simulink model "FCW_ROS_V1"  (R2022a)
settings: Solver=ode1  StartTime=0.0  StopTime=50  FixedStep=1  RelTol=1e-3
undefined symbols (not defined in the file): ACC, sigbuilder_block, speedController
libraries: slpidlib x5, simulink x2, robotlib x2
settings Model: NumberOfSteps=10  Creator=Kunj Patel  LastModifiedBy=dorleco
settings SolverCC: AlgebraicLoopSolver=TrustRegion
settings DebuggingCC: UnconnectedInputMsg=warning  UnconnectedOutputMsg=warning  UnconnectedLineMsg=warning  SFMachineParentedDataDiag=warning
settings SFSimCC: SimParseCustomCode=off
settings RTWCC: DLArmComputeVersion=19.05

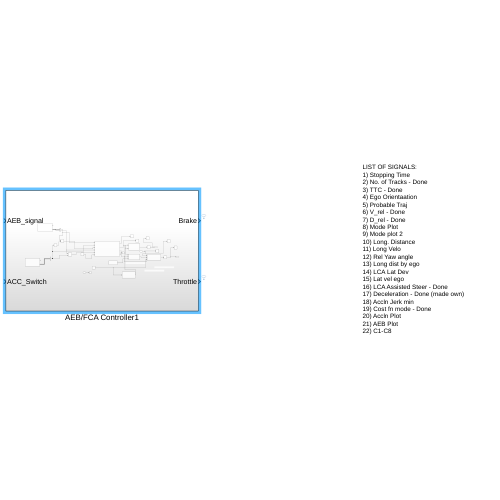
[thumbnail: Simulink's stored preview of the top-level diagram]
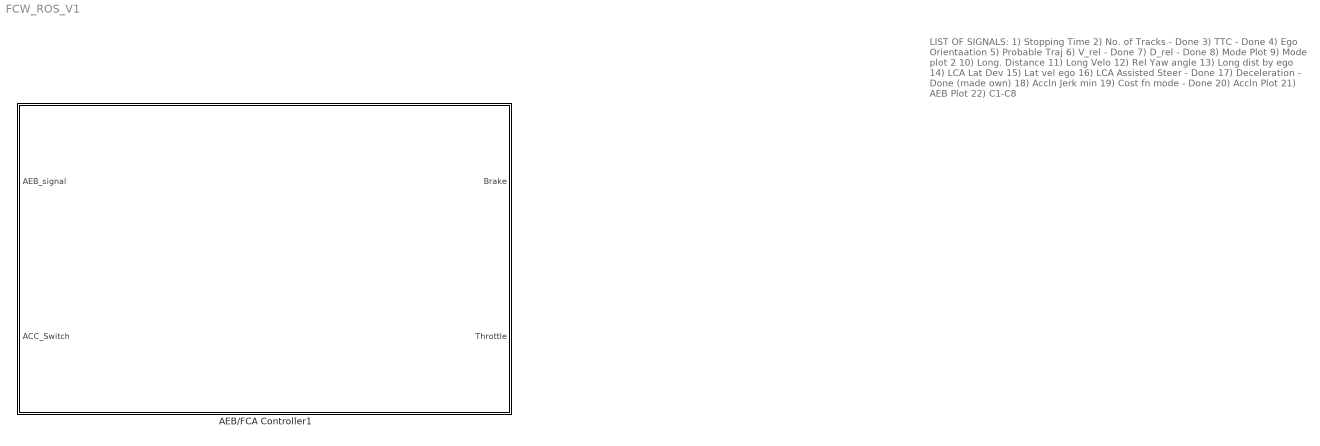
== system FCW_ROS_V1 ==
  note: LIST OF SIGNALS:
      | 1) Stopping Time
      | 2) No. of Tracks - Done
      | 3) TTC - Done
      | 4) Ego Orientaation
      | 5) Probable Traj
      | 6) V_rel - Done
      | 7) D_rel - Done
      | 8) Mode Plot
      | 9) Mode plot 2
      | 10) Long. Distance
      | 11) Long Velo
      | 12) Rel Yaw angle
      | 13) Long dist by ego
      | 14) LCA Lat Dev
      | 15) Lat vel ego
      | 16) LCA Assisted Steer - Done
      | 17) Deceleration - Done (made own)
      | 18) Accln Jerk min
      | 19) Cost fn mode - Done
      | 20) Accln Plot
      | 21) AEB Plot
      | 22) C1-C8
  AEB/FCA Controller1 : Subsystem

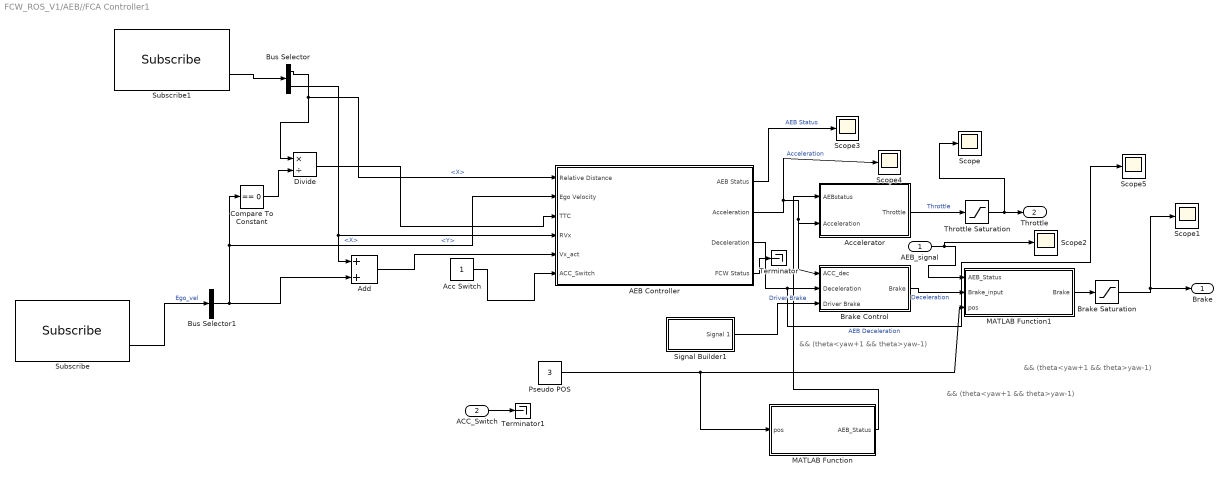
== system FCW_ROS_V1/AEB//FCA Controller1 ==
  note: && (theta<yaw+1 && theta>yaw-1)
  note: && (theta<yaw+1 && theta>yaw-1)
  note: && (theta<yaw+1 && theta>yaw-1)
  AEB_signal : Inport
  ACC_Switch : Inport  Port=2
  AEB Controller : Subsystem
  Acc Switch : Constant
  Accelerator : Subsystem
  Add : Sum
  Brake Control : Subsystem
  Brake Saturation : Saturate  UpperLimit=8  LowerLimit=0
  Bus Selector : BusSelector  OutputSignals=X,Y
  Bus Selector1 : BusSelector  OutputSignals=Twist.Twist.Linear.X
  Compare To Constant : simulink/Logic and Bit Operations/Compare To Constant  relop===  const=0  OutDataTypeStr=boolean
  Divide : Product  Inputs=*/
  MATLAB Function : MATLAB Function  TreatAsAtomicUnit=on
  MATLAB Function1 : MATLAB Function  TreatAsAtomicUnit=on
  Pseudo POS : Constant  Value=3
  Scope{,1..5} (6 alike) : Scope
  Signal Builder1 : Subsystem  Tag=STV Subsys  LoadFcn=sigbuilder_block('load');  StartFcn=sigbuilder_block('start');  StopFcn=sigbuilder_block('stop');  ClipboardFcn=sigbuilder_block('clipboard');  mask(Sigbuilder block){tuvar=[0:10]}
      mask help: Simulink:masks:SigbuilderBlock_MD
      mask init:
      | if ~strcmp(get_param(bdroot(gcbh),'SimulationStatus'),'stopped') tuvar = sigbuilder_block('maskInit'); end
      settings: CopyFcn=sigbuilder_block('copy');  DeleteFcn=sigbuilder_block('delete');  ModelCloseFcn=sigbuilder_block('modelClose');  PreSaveFcn=sigbuilder_block('preSave');  PauseFcn=sigbuilder_block('pause');  ContinueFcn=sigbuilder_block('continue');  NameChangeFcn=sigbuilder_block('namechange');  OpenFcn=sigbuilder_block('open',[302 88 550.5 362.5 ]);  CloseFcn=sigbuilder_block('close');
      mask Display: plot(0, 0, 100, 100,[2, 2, 32, 32, 2], [68, 8, 8, 68, 68],[32, 2], [38, 38], [32, 19, 2],[53, 60, 44], [32, 17, 17, 2],[16, 16, 31, 31]);txt = getActiveGroup(gcbh);text(2, 100, txt,'verticalAlignment', 'top');
  Subscribe : robotlib/Subscribe  topicSource=Select from ROS network  topic=/carla/ego_vehicle/odometry  messageType=nav_msgs/Odometry  SampleTime=1  legacyBusStruct=off  messageQueueLength=1
  Subscribe1 : robotlib/Subscribe  topicSource=Select from ROS network  topic=/perception/FCW  messageType=geometry_msgs/Point  SampleTime=1  legacyBusStruct=off  messageQueueLength=1
  Terminator : Terminator
  Terminator1 : Terminator
  Throttle Saturation : Saturate  UpperLimit=1.3  LowerLimit=0
  Brake : Outport
  Throttle : Outport  Port=2
  wires:
  Signal Builder1/1(Signal 1) -> Brake Control/3(Driver Brake)  "Driver Brake"
  AEB Controller/3(Deceleration) -> Scope5/1, Brake Control/2(Deceleration)  "AEB Deceleration"
  Accelerator/1(Throttle) -> Throttle Saturation/1  "Throttle"
  Throttle Saturation/1 -> Scope/1, Throttle/1
  Brake Saturation/1 -> Scope1/1, Brake/1
  AEB Controller/2(Acceleration) -> Scope4/1, Brake Control/1(ACC_dec), Accelerator/2(Acceleration)  "Acceleration"
  Divide/1 -> AEB Controller/3(TTC)
  AEB Controller/4(FCW Status) -> Terminator/1
  MATLAB Function1/1(Brake) -> Brake Saturation/1
  Brake Control/1(Brake) -> MATLAB Function1/2(Brake_input)  "Deceleration"
  AEB_signal/1 -> MATLAB Function1/1(AEB_Status), Scope2/1
  AEB Controller/1(AEB Status) -> Scope3/1  "AEB Status"
  MATLAB Function/1(AEB_Status) -> Accelerator/1(AEBstatus)
  ACC_Switch/1 -> Terminator1/1
  Acc Switch/1 -> AEB Controller/6(ACC_Switch)
  Pseudo POS/1 -> MATLAB Function1/3(pos), MATLAB Function/1(pos)
  Subscribe1/2 -> Bus Selector/1
  Subscribe/2 -> Bus Selector1/1  "Ego_vel"
  Bus Selector/1 -> AEB Controller/1(Relative Distance), Divide/1  "<X>"
  Bus Selector1/1 -> AEB Controller/2(Ego Velocity), Compare To Constant/1, Add/2  "<X>"
  Bus Selector/2 -> Add/1, AEB Controller/4(RVx)  "<Y>"
  Add/1 -> AEB Controller/5(Vx_act)
  Compare To Constant/1 -> Divide/2

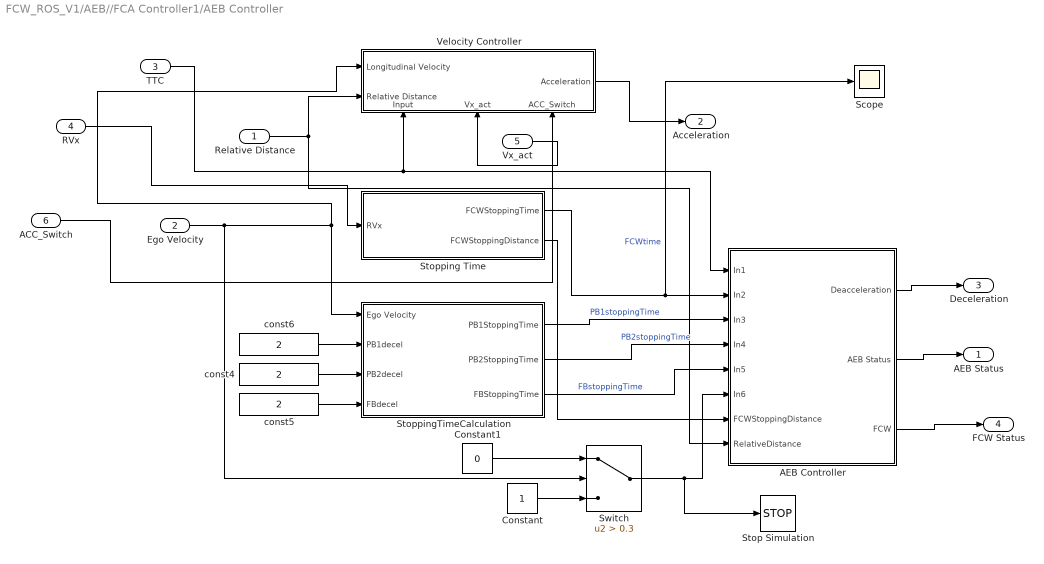
== system FCW_ROS_V1/AEB//FCA Controller1/AEB Controller ==
  Relative Distance : Inport
  Ego Velocity : Inport  Port=2
  TTC : Inport  Port=3
  RVx : Inport  Port=4
  Vx_act : Inport  Port=5
  ACC_Switch : Inport  Port=6
  AEB Controller : Subsystem
  Constant : Constant
  Constant1 : Constant  Value=0
  Scope : Scope
  Stop Simulation : Stop
  Stopping Time : Subsystem
  StoppingTimeCalculation : Subsystem
  Switch : Switch  Criteria=u2 > Threshold  Threshold=0.3  SaturateOnIntegerOverflow=off  InputSameDT=off
  Velocity Controller : Subsystem
      settings: PortSchema="{\"entries\":[{\"content\":{\"sides\":[{\"content\":{\"connectorIds\":[\"In1\",\"In2\"]},\"type\":\"ConnectorPlacement.EquallySpacedRectSide\",\"uuid\":\"796c06ee-5e3e-4c70-89bb-3872b2b2fec3\"},{\"content\":{\"connectorIds\":[\"Out1\"],\"side\":\"RIGHT\"},\"type\":\"ConnectorPlacement.EquallySpacedRectSide\",\"uuid\":\"23e41fbd-8b20-4aaf-a094-11b66cab9187\"},{\"content\":{\"connectorIds\":[],\"side\":\"TOP\"},\"type\":\"ConnectorPlacement.EquallySpacedRectSide\",\"uuid\":\"26342e9d-9e9e-43cc-a4c5-bfbf2895aede\"},{\"content\":{\"connectorIds\":[\"In3\",\"In4\",\"In5\"],\"side\":\"BOTTOM\"},\"type\":\"ConnectorPlacement.EquallySpacedRectSide\",\"uuid\":\"03d34232-b2fb-4d0e-a887-0a4704da0eeb\"}]},\"type\":\"ConnectorPlacement.EquallySpacedConnector\",\"uuid\":\"68d7bb64-97bc-4384-b049-e1fd777b4ed3\"}],\"packageUris\":[\"http://schema.mathworks.com/mf0/Connector/R2020b\"],\"version\":\"1.0\"}"
  const4 : Constant  Value=2  SampleTime=-1
  const5 : Constant  Value=2  SampleTime=-1
  const6 : Constant  Value=2  SampleTime=-1
  AEB Status : Outport  VectorParamsAs1DForOutWhenUnconnected=off
  Acceleration : Outport  Port=2  VectorParamsAs1DForOutWhenUnconnected=off
  Deceleration : Outport  Port=3  VectorParamsAs1DForOutWhenUnconnected=off
  FCW Status : Outport  Port=4  VectorParamsAs1DForOutWhenUnconnected=off
  wires:
  Relative Distance/1 -> AEB Controller/8(RelativeDistance), Velocity Controller/2(Relative Distance)
  const5/1 -> StoppingTimeCalculation/4(FBdecel)
  Stopping Time/1(FCWStoppingTime) -> Scope/1, AEB Controller/2(In2)  "FCWtime"
  const4/1 -> StoppingTimeCalculation/3(PB2decel)
  const6/1 -> StoppingTimeCalculation/2(PB1decel)
  Velocity Controller/1(Acceleration) -> Acceleration/1
  AEB Controller/2(AEB Status) -> AEB Status/1
  AEB Controller/1(Deacceleration) -> Deceleration/1
  AEB Controller/3(FCW) -> FCW Status/1
  StoppingTimeCalculation/3(FBStoppingTime) -> AEB Controller/5(In5)  "FBstoppingTime"
  StoppingTimeCalculation/2(PB2StoppingTime) -> AEB Controller/4(In4)  "PB2stoppingTime"
  StoppingTimeCalculation/1(PB1StoppingTime) -> AEB Controller/3(In3)  "PB1stoppingTime"
  TTC/1 -> AEB Controller/1(In1), Velocity Controller/3(Input)
  Ego Velocity/1 -> Switch/2, Velocity Controller/1(Longitudinal Velocity), StoppingTimeCalculation/1(Ego Velocity)
  Constant1/1 -> Switch/1
  Constant/1 -> Switch/3
  Switch/1 -> Stop Simulation/1, AEB Controller/6(In6)
  RVx/1 -> Stopping Time/1(RVx)
  Stopping Time/2(FCWStoppingDistance) -> AEB Controller/7(FCWStoppingDistance)
  Vx_act/1 -> Velocity Controller/4(Vx_act)
  ACC_Switch/1 -> Velocity Controller/5(ACC_Switch)

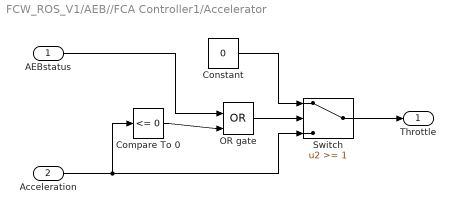
== system FCW_ROS_V1/AEB//FCA Controller1/Accelerator ==
  AEBstatus : Inport
  Acceleration : Inport  Port=2
  Compare To 0 : simulink/Logic and Bit Operations/Compare To Constant  relop=<=  const=0  OutDataTypeStr=boolean
  Constant : Constant  Value=0
  OR gate : Logic  Operator=OR  IconShape=distinctive  AllPortsSameDT=off  OutDataTypeStr=boolean
  "Switch " : Switch  Threshold=1  SaturateOnIntegerOverflow=off  InputSameDT=off
  Throttle : Outport  VectorParamsAs1DForOutWhenUnconnected=off
  wires:
  "Switch "/1 -> Throttle/1
  Constant/1 -> "Switch "/1
  Acceleration/1 -> Compare To 0/1, "Switch "/3
  AEBstatus/1 -> OR gate/1
  OR gate/1 -> "Switch "/2
  Compare To 0/1 -> OR gate/2

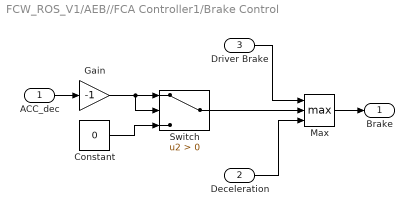
== system FCW_ROS_V1/AEB//FCA Controller1/Brake Control ==
  ACC_dec : Inport
  Deceleration : Inport  Port=2
  Driver Brake : Inport  Port=3
  Constant : Constant  Value=0
  Gain : Gain  Gain=-1
  Max : MinMax  Function=max  Inputs=3
  "Switch " : Switch  Criteria=u2 > Threshold  SaturateOnIntegerOverflow=off  InputSameDT=off
  Brake : Outport  VectorParamsAs1DForOutWhenUnconnected=off
  wires:
  Max/1 -> Brake/1
  Driver Brake/1 -> Max/1
  Deceleration/1 -> Max/3
  "Switch "/1 -> Max/2
  ACC_dec/1 -> Gain/1
  Gain/1 -> "Switch "/2, "Switch "/1
  Constant/1 -> "Switch "/3

== system FCW_ROS_V1/AEB//FCA Controller1/Signal Builder1 ==
  Demux : Demux  Tag=STV Demux  Outputs=1
      settings: DisplayOption=none
  FromWs : FromWorkspace  Tag=STV FromWs  VariableName=tuvar
      SigBuilderData=|
      | common.afterFinalStr = 'Extrapolate'
      | common.sampleTime = 0
      | dataSet.timeRange = [0 20]
      | dataSet.name = 'Group 1'
      | sbobj.Groups.Name = 'Group 1'
      | sbobj.Groups.Signals.Name = 'Signal 1'
      | sbobj.Groups.Signals.XData = [0 20]
      | sbobj.Groups.Signals.YData = [0 0]
      | sbobj.Groups.TimeRange = [0 20]
  Signal 1 : Outport  Tag=STV Outport  VectorParamsAs1DForOutWhenUnconnected=off
  wires:
  FromWs/1 -> Demux/1
  Demux/1 -> Signal 1/1

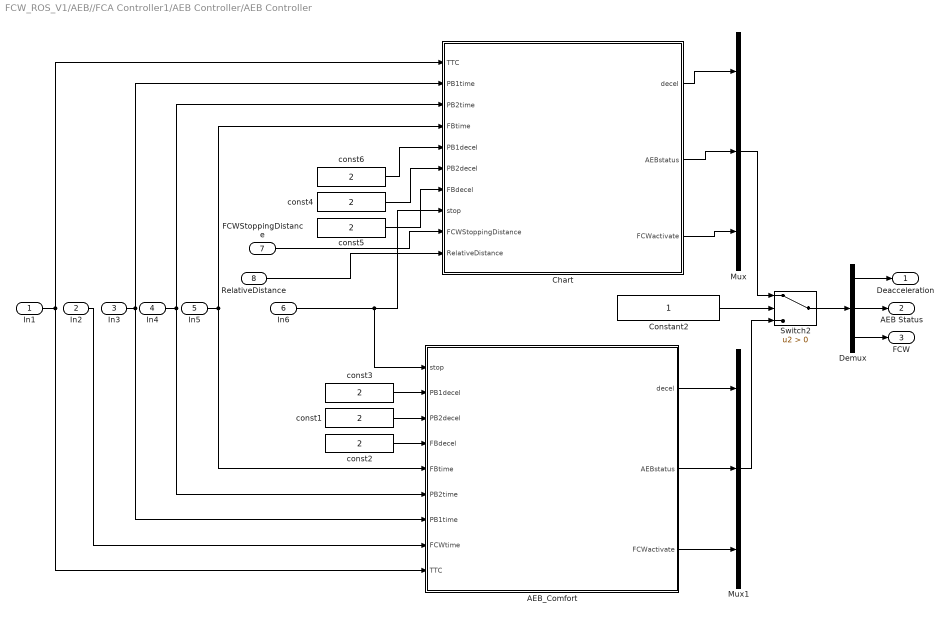
== system FCW_ROS_V1/AEB//FCA Controller1/AEB Controller/AEB Controller ==
  In1 : Inport
  In2 : Inport  Port=2
  In3 : Inport  Port=3
  In4 : Inport  Port=4
  In5 : Inport  Port=5
  In6 : Inport  Port=6
  FCWStoppingDistance : Inport  Port=7
  RelativeDistance : Inport  Port=8
  AEB_Comfort : Stateflow chart  TreatAsAtomicUnit=on
  Chart : Stateflow chart  TreatAsAtomicUnit=on
  Constant2 : Constant
  Demux : Demux  Outputs=3
  Mux : Mux  Inputs=3
  Mux1 : Mux  Inputs=3
  Switch2 : Switch  Criteria=u2 > Threshold  SaturateOnIntegerOverflow=off  InputSameDT=off
  const{1..6} (6 alike) : Constant  Value=2  SampleTime=-1
  Deacceleration : Outport  VectorParamsAs1DForOutWhenUnconnected=off
  AEB Status : Outport  Port=2  VectorParamsAs1DForOutWhenUnconnected=off
  FCW : Outport  Port=3  VectorParamsAs1DForOutWhenUnconnected=off
  wires:
  In6/1 -> AEB_Comfort/1(stop), Chart/8(stop)
  In1/1 -> AEB_Comfort/9(TTC), Chart/1(TTC)
  Chart/2(AEBstatus) -> Mux/2
  const1/1 -> AEB_Comfort/3(PB2decel)
  Constant2/1 -> Switch2/2
  const3/1 -> AEB_Comfort/2(PB1decel)
  Mux/1 -> Switch2/1
  Switch2/1 -> Demux/1
  In4/1 -> AEB_Comfort/6(PB2time), Chart/3(PB2time)
  In5/1 -> AEB_Comfort/5(FBtime), Chart/4(FBtime)
  const2/1 -> AEB_Comfort/4(FBdecel)
  Mux1/1 -> Switch2/3
  Demux/3 -> FCW/1
  In2/1 -> AEB_Comfort/8(FCWtime)
  Demux/2 -> AEB Status/1
  Demux/1 -> Deacceleration/1
  In3/1 -> AEB_Comfort/7(PB1time), Chart/2(PB1time)
  Chart/1(decel) -> Mux/1
  Chart/3(FCWactivate) -> Mux/3
  const6/1 -> Chart/5(PB1decel)
  const4/1 -> Chart/6(PB2decel)
  const5/1 -> Chart/7(FBdecel)
  AEB_Comfort/1(decel) -> Mux1/1
  AEB_Comfort/2(AEBstatus) -> Mux1/2
  AEB_Comfort/3(FCWactivate) -> Mux1/3
  FCWStoppingDistance/1 -> Chart/9(FCWStoppingDistance)
  RelativeDistance/1 -> Chart/10(RelativeDistance)

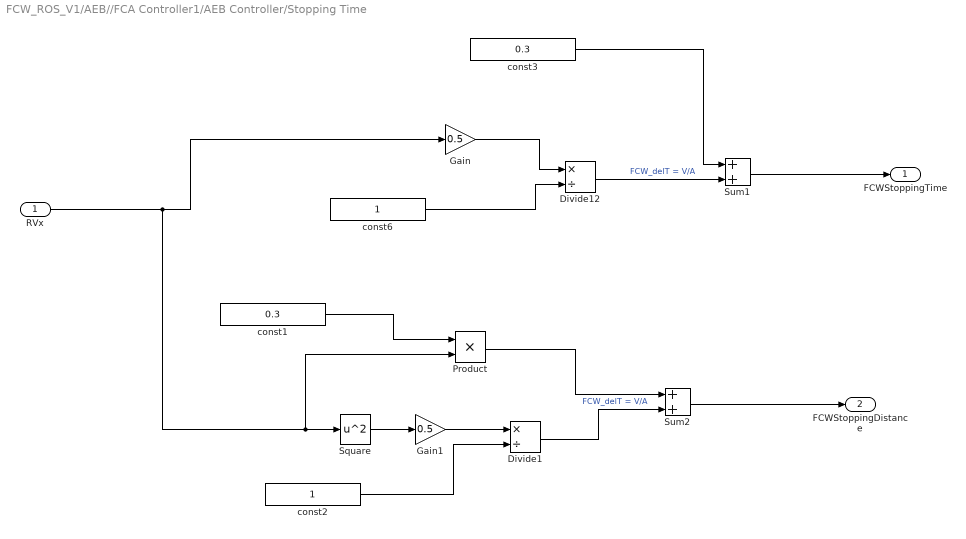
== system FCW_ROS_V1/AEB//FCA Controller1/AEB Controller/Stopping Time ==
  RVx : Inport
  Divide1 : Product  Inputs=*/
  Divide12 : Product  Inputs=*/
  Gain : Gain  Gain=0.5
  Gain1 : Gain  Gain=0.5
  Product : Product
  Square : Math  Operator=square
  Sum1 : Sum
  Sum2 : Sum
  const1 : Constant  Value=0.3  SampleTime=-1
  const2 : Constant  SampleTime=-1
  const3 : Constant  Value=0.3  SampleTime=-1
  const6 : Constant  SampleTime=-1
  FCWStoppingTime : Outport  VectorParamsAs1DForOutWhenUnconnected=off
  FCWStoppingDistance : Outport  Port=2  VectorParamsAs1DForOutWhenUnconnected=off
  wires:
  const3/1 -> Sum1/1
  const6/1 -> Divide12/2
  Sum1/1 -> FCWStoppingTime/1
  Divide12/1 -> Sum1/2  "FCW_delT = V/A"
  Gain/1 -> Divide12/1
  Sum2/1 -> FCWStoppingDistance/1
  RVx/1 -> Product/2, Square/1, Gain/1
  Gain1/1 -> Divide1/1
  Divide1/1 -> Sum2/2  "FCW_delT = V/A"
  const2/1 -> Divide1/2
  const1/1 -> Product/1
  Product/1 -> Sum2/1
  Square/1 -> Gain1/1

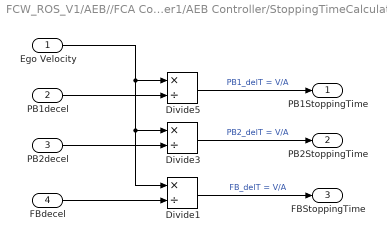
== system FCW_ROS_V1/AEB//FCA Controller1/AEB Controller/StoppingTimeCalculation ==
  Ego Velocity : Inport
  PB1decel : Inport  Port=2
  PB2decel : Inport  Port=3
  FBdecel : Inport  Port=4
  Divide1 : Product  Inputs=*/
  Divide3 : Product  Inputs=*/
  Divide5 : Product  Inputs=*/
  PB1StoppingTime : Outport  VectorParamsAs1DForOutWhenUnconnected=off
  PB2StoppingTime : Outport  Port=2  VectorParamsAs1DForOutWhenUnconnected=off
  FBStoppingTime : Outport  Port=3  VectorParamsAs1DForOutWhenUnconnected=off
  wires:
  Divide5/1 -> PB1StoppingTime/1  "PB1_delT = V/A"
  Divide3/1 -> PB2StoppingTime/1  "PB2_delT = V/A"
  Divide1/1 -> FBStoppingTime/1  "FB_delT = V/A"
  PB1decel/1 -> Divide5/2
  PB2decel/1 -> Divide3/2
  FBdecel/1 -> Divide1/2
  Ego Velocity/1 -> Divide1/1, Divide3/1, Divide5/1

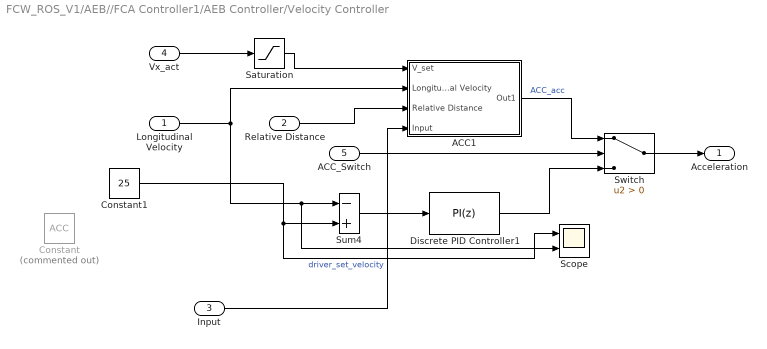
== system FCW_ROS_V1/AEB//FCA Controller1/AEB Controller/Velocity Controller ==
  Longitudinal Velocity : Inport
  Relative Distance : Inport  Port=2
  Input : Inport  Port=3
  Vx_act : Inport  Port=4
  ACC_Switch : Inport  Port=5
  ACC1 : Subsystem
  Constant : Constant  Commented=on  Value=ACC
  Constant1 : Constant  Value=25
  Discrete PID Controller1 : slpidlib/PID Controller  Controller=PI  Form=Parallel  TimeDomain=Discrete-time  UseExternalTs=off  SampleTime=-1  IntegratorMethod=Forward Euler  FilterMethod=Forward Euler  ControllerParametersSource=internal  P=10  I=4  UseKiTs=off  D=speedController.Kd  N=speedController.FilterCoeff  UseFilter=on  TunerSelectOption=Transfer Function Based (PID Tuner App)  InitialConditionSource=internal  InitialConditionForIntegrator=0  InitialConditionForFilter=0  DifferentiatorICPrevScaledInput=0  ExternalReset=none  TrackingMode=off  Kt=1  LimitOutput=on  SatLimitsSource=internal  UpperSaturationLimit=5  LowerSaturationLimit=-5  LinearizeAsGain=off  AntiWindupMode=clamping  Kb=1  POutMin=[]  POutMax=[]  IOutMin=[]  IOutMax=[]  DOutMin=[]  DOutMax=[]  NOutMin=[]  NOutMax=[]  SumOutMin=[]  SumOutMax=[]  SaturationOutMin=[]  SaturationOutMax=[]  PParamMin=[]  PParamMax=[]  IParamMin=[]  IParamMax=[]  DParamMin=[]  DParamMax=[]  NParamMin=[]  NParamMax=[]  KbParamMin=[]  KbParamMax=[]  KtParamMin=[]  KtParamMax=[]  KbOutMin=[]  KbOutMax=[]  KtOutMin=[]  KtOutMax=[]  IntegratorOutMin=[]  IntegratorOutMax=[]  FilterOutMin=[]  FilterOutMax=[]  SumI1OutMin=[]  SumI1OutMax=[]  SumI2OutMin=[]  SumI2OutMax=[]  SumI3OutMin=[]  SumI3OutMax=[]  SumI4OutMin=[]  SumI4OutMax=[]  SumDOutMin=[]  SumDOutMax=[]  DifferentiatorOutMin=[]  DifferentiatorOutMax=[]  FilterDiffOutCoefMin=[]  FilterDiffOutCoefMax=[]  ReciprocalOutMin=[]  ReciprocalOutMax=[]  SumDenOutMin=[]  SumDenOutMax=[]  SumNumOutMin=[]  SumNumOutMax=[]  DivideOutMin=[]  DivideOutMax=[]  UdiffTsProdOutMin=[]  UdiffTsProdOutMax=[]  NTsProdOutMin=[]  NTsProdOutMax=[]  UintegralTsProdOutMin=[]  UintegralTsProdOutMax=[]  UngainTsProdOutMin=[]  UngainTsProdOutMax=[]  IntegratorContinuousStateAttributes=''  IntegratorStateMustResolveToSignalObject=off  IntegratorRTWStateStorageClass=Auto  FilterContinuousStateAttributes=''  FilterStateMustResolveToSignalObject=off  FilterRTWStateStorageClass=Auto  ParallelPVariant=InternalParameters  IdealPVariant=Disabled  IVariant=InternalParameters  DVariant=Disabled  IntegratorVariant=Discrete  SatVariant=Enabled  AWVariant=DiscClampingParallel  PCopyVariant=Disabled  TRVariant=Disabled  FdbkBlocksVariant=Forward  IdealPFdbkVariant=Disabled  SatFdbkVariant=Disabled  DerivativeFilterVariant=Disabled  NVariant=Disabled  NCopyVariant=Disabled_SignalSpec  FilterICVariant=Disabled  IntegratorICVariant=InternalICs  ExternalResetVariant=Disabled  TRSumVariant=Passthrough  SumFdbkVariant=Disabled  SumVariant=Sum_PI  TsampFilterVariant=InternalTs  TsampNgainVariant=Passthrough  TsampIntegralVariant=Passthrough  ExternalSaturationOutDataTypeStr=Inherit: Same as second input  aMode=0
  Saturation : Saturate  UpperLimit=30  LowerLimit=-100
  Scope : Scope  NumInputPorts=2
  Sum4 : Sum  Inputs=-+
  Switch : Switch  Criteria=u2 > Threshold  SaturateOnIntegerOverflow=off  InputSameDT=off
  Acceleration : Outport  VectorParamsAs1DForOutWhenUnconnected=off
  wires:
  Sum4/1 -> Discrete PID Controller1/1
  ACC_Switch/1 -> Switch/2
  Constant1/1 -> Scope/1, Sum4/2  "driver_set_velocity"
  Switch/1 -> Acceleration/1
  Discrete PID Controller1/1 -> Switch/3
  Longitudinal Velocity/1 -> ACC1/2(Longitudinal Velocity), Scope/2, Sum4/1
  Relative Distance/1 -> ACC1/3(Relative Distance)
  ACC1/1(Out1) -> Switch/1  "ACC_acc"
  Input/1 -> ACC1/4(Input)
  Vx_act/1 -> Saturation/1
  Saturation/1 -> ACC1/1(V_set)

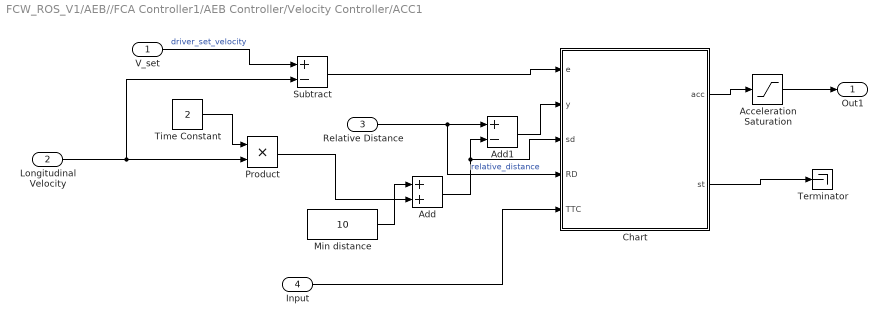
== system FCW_ROS_V1/AEB//FCA Controller1/AEB Controller/Velocity Controller/ACC1 ==
  V_set : Inport
  Longitudinal Velocity : Inport  Port=2
  Relative Distance : Inport  Port=3
  Input : Inport  Port=4
  Acceleration Saturation : Saturate  UpperLimit=1.3  LowerLimit=-1.3
  Add : Sum
  Add1 : Sum  Inputs=+-
  Chart : Stateflow chart  TreatAsAtomicUnit=on
  Min distance : Constant  Value=10
  Product : Product
  Subtract : Sum  Inputs=+-
  Terminator : Terminator
  Time Constant : Constant  Value=2
  Out1 : Outport
  wires:
  Time Constant/1 -> Product/1
  Longitudinal Velocity/1 -> Subtract/2, Product/2
  Chart/1(acc) -> Acceleration Saturation/1
  Min distance/1 -> Add/1
  Product/1 -> Add/2
  Acceleration Saturation/1 -> Out1/1
  Chart/2(st) -> Terminator/1
  Add/1 -> Chart/3(sd), Add1/2
  Relative Distance/1 -> Chart/4(RD), Add1/1  "relative_distance"
  Add1/1 -> Chart/2(y)
  V_set/1 -> Subtract/1  "driver_set_velocity"
  Subtract/1 -> Chart/1(e)
  Input/1 -> Chart/5(TTC)

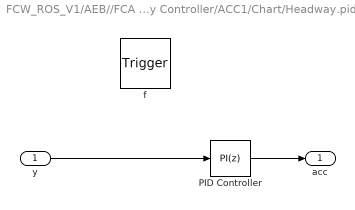
== system FCW_ROS_V1/AEB//FCA Controller1/AEB Controller/Velocity Controller/ACC1/Chart/Headway.pid_control ==
  y : Inport  OutDataTypeStr=double  PortDimensions=1
  f : TriggerPort  TriggerType=function-call  VariantControl=(inherit)
      settings: CopyFcn=Stateflow.SLINSF.SimulinkMan.removeBlockPreDeleteFcn  PreDeleteFcn=Stateflow.SLINSF.SimulinkMan.unsafePredeleteFcn
  PID Controller : slpidlib/PID Controller  Controller=PI  Form=Parallel  TimeDomain=Discrete-time  UseExternalTs=off  SampleTime=-1  IntegratorMethod=Forward Euler  FilterMethod=Forward Euler  ControllerParametersSource=internal  P=12  I=0  UseKiTs=off  D=0  N=100  UseFilter=on  TunerSelectOption=Transfer Function Based (PID Tuner App)  InitialConditionSource=internal  InitialConditionForIntegrator=0  InitialConditionForFilter=0  DifferentiatorICPrevScaledInput=0  ExternalReset=none  TrackingMode=off  Kt=1  LimitOutput=off  SatLimitsSource=internal  UpperSaturationLimit=inf  LowerSaturationLimit=-inf  LinearizeAsGain=on  AntiWindupMode=none  Kb=1  POutMin=[]  POutMax=[]  IOutMin=[]  IOutMax=[]  DOutMin=[]  DOutMax=[]  NOutMin=[]  NOutMax=[]  SumOutMin=[]  SumOutMax=[]  SaturationOutMin=[]  SaturationOutMax=[]  PParamMin=[]  PParamMax=[]  IParamMin=[]  IParamMax=[]  DParamMin=[]  DParamMax=[]  NParamMin=[]  NParamMax=[]  KbParamMin=[]  KbParamMax=[]  KtParamMin=[]  KtParamMax=[]  KbOutMin=[]  KbOutMax=[]  KtOutMin=[]  KtOutMax=[]  IntegratorOutMin=[]  IntegratorOutMax=[]  FilterOutMin=[]  FilterOutMax=[]  SumI1OutMin=[]  SumI1OutMax=[]  SumI2OutMin=[]  SumI2OutMax=[]  SumI3OutMin=[]  SumI3OutMax=[]  SumI4OutMin=[]  SumI4OutMax=[]  SumDOutMin=[]  SumDOutMax=[]  DifferentiatorOutMin=[]  DifferentiatorOutMax=[]  FilterDiffOutCoefMin=[]  FilterDiffOutCoefMax=[]  ReciprocalOutMin=[]  ReciprocalOutMax=[]  SumDenOutMin=[]  SumDenOutMax=[]  SumNumOutMin=[]  SumNumOutMax=[]  DivideOutMin=[]  DivideOutMax=[]  UdiffTsProdOutMin=[]  UdiffTsProdOutMax=[]  NTsProdOutMin=[]  NTsProdOutMax=[]  UintegralTsProdOutMin=[]  UintegralTsProdOutMax=[]  UngainTsProdOutMin=[]  UngainTsProdOutMax=[]  IntegratorContinuousStateAttributes=''  IntegratorStateMustResolveToSignalObject=off  IntegratorRTWStateStorageClass=Auto  FilterContinuousStateAttributes=''  FilterStateMustResolveToSignalObject=off  FilterRTWStateStorageClass=Auto  ParallelPVariant=InternalParameters  IdealPVariant=Disabled  IVariant=InternalParameters  DVariant=Disabled  IntegratorVariant=Discrete  SatVariant=Disabled  AWVariant=Passthrough  PCopyVariant=Disabled  TRVariant=Disabled  FdbkBlocksVariant=Forward  IdealPFdbkVariant=Disabled  SatFdbkVariant=Disabled  DerivativeFilterVariant=Disabled  NVariant=Disabled  NCopyVariant=Disabled_SignalSpec  FilterICVariant=Disabled  IntegratorICVariant=InternalICs  ExternalResetVariant=Disabled  TRSumVariant=Passthrough  SumFdbkVariant=Disabled  SumVariant=Sum_PI  TsampFilterVariant=InternalTs  TsampNgainVariant=Passthrough  TsampIntegralVariant=Passthrough  ExternalSaturationOutDataTypeStr=Inherit: Same as second input  aMode=0
  acc : Outport
  wires:
  PID Controller/1 -> acc/1
  y/1 -> PID Controller/1

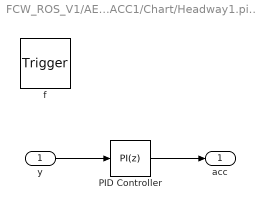
== system FCW_ROS_V1/AEB//FCA Controller1/AEB Controller/Velocity Controller/ACC1/Chart/Headway1.pid_control ==
  y : Inport  OutDataTypeStr=double  PortDimensions=1
  f : TriggerPort  TriggerType=function-call  VariantControl=(inherit)
      settings: CopyFcn=Stateflow.SLINSF.SimulinkMan.removeBlockPreDeleteFcn  PreDeleteFcn=Stateflow.SLINSF.SimulinkMan.unsafePredeleteFcn
  PID Controller : slpidlib/PID Controller  Controller=PI  Form=Parallel  TimeDomain=Discrete-time  UseExternalTs=off  SampleTime=-1  IntegratorMethod=Forward Euler  FilterMethod=Forward Euler  ControllerParametersSource=internal  P=12  I=0  UseKiTs=off  D=0  N=100  UseFilter=on  TunerSelectOption=Transfer Function Based (PID Tuner App)  InitialConditionSource=internal  InitialConditionForIntegrator=0  InitialConditionForFilter=0  DifferentiatorICPrevScaledInput=0  ExternalReset=none  TrackingMode=off  Kt=1  LimitOutput=off  SatLimitsSource=internal  UpperSaturationLimit=inf  LowerSaturationLimit=-inf  LinearizeAsGain=on  AntiWindupMode=none  Kb=1  POutMin=[]  POutMax=[]  IOutMin=[]  IOutMax=[]  DOutMin=[]  DOutMax=[]  NOutMin=[]  NOutMax=[]  SumOutMin=[]  SumOutMax=[]  SaturationOutMin=[]  SaturationOutMax=[]  PParamMin=[]  PParamMax=[]  IParamMin=[]  IParamMax=[]  DParamMin=[]  DParamMax=[]  NParamMin=[]  NParamMax=[]  KbParamMin=[]  KbParamMax=[]  KtParamMin=[]  KtParamMax=[]  KbOutMin=[]  KbOutMax=[]  KtOutMin=[]  KtOutMax=[]  IntegratorOutMin=[]  IntegratorOutMax=[]  FilterOutMin=[]  FilterOutMax=[]  SumI1OutMin=[]  SumI1OutMax=[]  SumI2OutMin=[]  SumI2OutMax=[]  SumI3OutMin=[]  SumI3OutMax=[]  SumI4OutMin=[]  SumI4OutMax=[]  SumDOutMin=[]  SumDOutMax=[]  DifferentiatorOutMin=[]  DifferentiatorOutMax=[]  FilterDiffOutCoefMin=[]  FilterDiffOutCoefMax=[]  ReciprocalOutMin=[]  ReciprocalOutMax=[]  SumDenOutMin=[]  SumDenOutMax=[]  SumNumOutMin=[]  SumNumOutMax=[]  DivideOutMin=[]  DivideOutMax=[]  UdiffTsProdOutMin=[]  UdiffTsProdOutMax=[]  NTsProdOutMin=[]  NTsProdOutMax=[]  UintegralTsProdOutMin=[]  UintegralTsProdOutMax=[]  UngainTsProdOutMin=[]  UngainTsProdOutMax=[]  IntegratorContinuousStateAttributes=''  IntegratorStateMustResolveToSignalObject=off  IntegratorRTWStateStorageClass=Auto  FilterContinuousStateAttributes=''  FilterStateMustResolveToSignalObject=off  FilterRTWStateStorageClass=Auto  ParallelPVariant=InternalParameters  IdealPVariant=Disabled  IVariant=InternalParameters  DVariant=Disabled  IntegratorVariant=Discrete  SatVariant=Disabled  AWVariant=Passthrough  PCopyVariant=Disabled  TRVariant=Disabled  FdbkBlocksVariant=Forward  IdealPFdbkVariant=Disabled  SatFdbkVariant=Disabled  DerivativeFilterVariant=Disabled  NVariant=Disabled  NCopyVariant=Disabled_SignalSpec  FilterICVariant=Disabled  IntegratorICVariant=InternalICs  ExternalResetVariant=Disabled  TRSumVariant=Passthrough  SumFdbkVariant=Disabled  SumVariant=Sum_PI  TsampFilterVariant=InternalTs  TsampNgainVariant=Passthrough  TsampIntegralVariant=Passthrough  ExternalSaturationOutDataTypeStr=Inherit: Same as second input  aMode=0
  acc : Outport
  wires:
  PID Controller/1 -> acc/1
  y/1 -> PID Controller/1

== system FCW_ROS_V1/AEB//FCA Controller1/AEB Controller/Velocity Controller/ACC1/Chart/Velocity.pid_control ==
  e : Inport  OutDataTypeStr=double  PortDimensions=1
  f : TriggerPort  TriggerType=function-call  VariantControl=(inherit)
      settings: CopyFcn=Stateflow.SLINSF.SimulinkMan.removeBlockPreDeleteFcn  PreDeleteFcn=Stateflow.SLINSF.SimulinkMan.unsafePredeleteFcn
  PID Controller : slpidlib/PID Controller  Controller=PI  Form=Parallel  TimeDomain=Discrete-time  UseExternalTs=off  SampleTime=-1  IntegratorMethod=Forward Euler  FilterMethod=Forward Euler  ControllerParametersSource=internal  P=4  I=0  UseKiTs=off  D=0  N=100  UseFilter=on  TunerSelectOption=Transfer Function Based (PID Tuner App)  InitialConditionSource=internal  InitialConditionForIntegrator=0  InitialConditionForFilter=0  DifferentiatorICPrevScaledInput=0  ExternalReset=none  TrackingMode=off  Kt=1  LimitOutput=off  SatLimitsSource=internal  UpperSaturationLimit=inf  LowerSaturationLimit=-inf  LinearizeAsGain=on  AntiWindupMode=none  Kb=1  POutMin=[]  POutMax=[]  IOutMin=[]  IOutMax=[]  DOutMin=[]  DOutMax=[]  NOutMin=[]  NOutMax=[]  SumOutMin=[]  SumOutMax=[]  SaturationOutMin=[]  SaturationOutMax=[]  PParamMin=[]  PParamMax=[]  IParamMin=[]  IParamMax=[]  DParamMin=[]  DParamMax=[]  NParamMin=[]  NParamMax=[]  KbParamMin=[]  KbParamMax=[]  KtParamMin=[]  KtParamMax=[]  KbOutMin=[]  KbOutMax=[]  KtOutMin=[]  KtOutMax=[]  IntegratorOutMin=[]  IntegratorOutMax=[]  FilterOutMin=[]  FilterOutMax=[]  SumI1OutMin=[]  SumI1OutMax=[]  SumI2OutMin=[]  SumI2OutMax=[]  SumI3OutMin=[]  SumI3OutMax=[]  SumI4OutMin=[]  SumI4OutMax=[]  SumDOutMin=[]  SumDOutMax=[]  DifferentiatorOutMin=[]  DifferentiatorOutMax=[]  FilterDiffOutCoefMin=[]  FilterDiffOutCoefMax=[]  ReciprocalOutMin=[]  ReciprocalOutMax=[]  SumDenOutMin=[]  SumDenOutMax=[]  SumNumOutMin=[]  SumNumOutMax=[]  DivideOutMin=[]  DivideOutMax=[]  UdiffTsProdOutMin=[]  UdiffTsProdOutMax=[]  NTsProdOutMin=[]  NTsProdOutMax=[]  UintegralTsProdOutMin=[]  UintegralTsProdOutMax=[]  UngainTsProdOutMin=[]  UngainTsProdOutMax=[]  IntegratorContinuousStateAttributes=''  IntegratorStateMustResolveToSignalObject=off  IntegratorRTWStateStorageClass=Auto  FilterContinuousStateAttributes=''  FilterStateMustResolveToSignalObject=off  FilterRTWStateStorageClass=Auto  ParallelPVariant=InternalParameters  IdealPVariant=Disabled  IVariant=InternalParameters  DVariant=Disabled  IntegratorVariant=Discrete  SatVariant=Disabled  AWVariant=Passthrough  PCopyVariant=Disabled  TRVariant=Disabled  FdbkBlocksVariant=Forward  IdealPFdbkVariant=Disabled  SatFdbkVariant=Disabled  DerivativeFilterVariant=Disabled  NVariant=Disabled  NCopyVariant=Disabled_SignalSpec  FilterICVariant=Disabled  IntegratorICVariant=InternalICs  ExternalResetVariant=Disabled  TRSumVariant=Passthrough  SumFdbkVariant=Disabled  SumVariant=Sum_PI  TsampFilterVariant=InternalTs  TsampNgainVariant=Passthrough  TsampIntegralVariant=Passthrough  ExternalSaturationOutDataTypeStr=Inherit: Same as second input  aMode=0
  acc : Outport
  wires:
  PID Controller/1 -> acc/1
  e/1 -> PID Controller/1

== system FCW_ROS_V1/AEB//FCA Controller1/AEB Controller/Velocity Controller/ACC1/Chart/Velocity1.pid_control ==
  e : Inport  OutDataTypeStr=double  PortDimensions=1
  f : TriggerPort  TriggerType=function-call  VariantControl=(inherit)
      settings: CopyFcn=Stateflow.SLINSF.SimulinkMan.removeBlockPreDeleteFcn  PreDeleteFcn=Stateflow.SLINSF.SimulinkMan.unsafePredeleteFcn
  PID Controller : slpidlib/PID Controller  Controller=PI  Form=Parallel  TimeDomain=Discrete-time  UseExternalTs=off  SampleTime=-1  IntegratorMethod=Forward Euler  FilterMethod=Forward Euler  ControllerParametersSource=internal  P=4  I=0  UseKiTs=off  D=0  N=100  UseFilter=on  TunerSelectOption=Transfer Function Based (PID Tuner App)  InitialConditionSource=internal  InitialConditionForIntegrator=0  InitialConditionForFilter=0  DifferentiatorICPrevScaledInput=0  ExternalReset=none  TrackingMode=off  Kt=1  LimitOutput=off  SatLimitsSource=internal  UpperSaturationLimit=inf  LowerSaturationLimit=-inf  LinearizeAsGain=on  AntiWindupMode=none  Kb=1  POutMin=[]  POutMax=[]  IOutMin=[]  IOutMax=[]  DOutMin=[]  DOutMax=[]  NOutMin=[]  NOutMax=[]  SumOutMin=[]  SumOutMax=[]  SaturationOutMin=[]  SaturationOutMax=[]  PParamMin=[]  PParamMax=[]  IParamMin=[]  IParamMax=[]  DParamMin=[]  DParamMax=[]  NParamMin=[]  NParamMax=[]  KbParamMin=[]  KbParamMax=[]  KtParamMin=[]  KtParamMax=[]  KbOutMin=[]  KbOutMax=[]  KtOutMin=[]  KtOutMax=[]  IntegratorOutMin=[]  IntegratorOutMax=[]  FilterOutMin=[]  FilterOutMax=[]  SumI1OutMin=[]  SumI1OutMax=[]  SumI2OutMin=[]  SumI2OutMax=[]  SumI3OutMin=[]  SumI3OutMax=[]  SumI4OutMin=[]  SumI4OutMax=[]  SumDOutMin=[]  SumDOutMax=[]  DifferentiatorOutMin=[]  DifferentiatorOutMax=[]  FilterDiffOutCoefMin=[]  FilterDiffOutCoefMax=[]  ReciprocalOutMin=[]  ReciprocalOutMax=[]  SumDenOutMin=[]  SumDenOutMax=[]  SumNumOutMin=[]  SumNumOutMax=[]  DivideOutMin=[]  DivideOutMax=[]  UdiffTsProdOutMin=[]  UdiffTsProdOutMax=[]  NTsProdOutMin=[]  NTsProdOutMax=[]  UintegralTsProdOutMin=[]  UintegralTsProdOutMax=[]  UngainTsProdOutMin=[]  UngainTsProdOutMax=[]  IntegratorContinuousStateAttributes=''  IntegratorStateMustResolveToSignalObject=off  IntegratorRTWStateStorageClass=Auto  FilterContinuousStateAttributes=''  FilterStateMustResolveToSignalObject=off  FilterRTWStateStorageClass=Auto  ParallelPVariant=InternalParameters  IdealPVariant=Disabled  IVariant=InternalParameters  DVariant=Disabled  IntegratorVariant=Discrete  SatVariant=Disabled  AWVariant=Passthrough  PCopyVariant=Disabled  TRVariant=Disabled  FdbkBlocksVariant=Forward  IdealPFdbkVariant=Disabled  SatFdbkVariant=Disabled  DerivativeFilterVariant=Disabled  NVariant=Disabled  NCopyVariant=Disabled_SignalSpec  FilterICVariant=Disabled  IntegratorICVariant=InternalICs  ExternalResetVariant=Disabled  TRSumVariant=Passthrough  SumFdbkVariant=Disabled  SumVariant=Sum_PI  TsampFilterVariant=InternalTs  TsampNgainVariant=Passthrough  TsampIntegralVariant=Passthrough  ExternalSaturationOutDataTypeStr=Inherit: Same as second input  aMode=0
  acc : Outport
  wires:
  PID Controller/1 -> acc/1
  e/1 -> PID Controller/1

== matlab function FCW_ROS_V1/AEB//FCA Controller1/MATLAB Function1 ==
  data: AEB_Status input; Brake output; Brake_input input; pos input
function Brake = fcn(AEB_Status,Brake_input,pos)
if AEB_Status == 0 || pos~=3
    Brake = 0;
else
    if abs(Brake_input)<3
        Brake = Brake_input + 2;
    else
        Brake = Brake_input;
    end
end
end

== matlab function FCW_ROS_V1/AEB//FCA Controller1/MATLAB Function ==
  data: pos input; AEB_Status output
function AEB_Status = fcn(pos)
if pos==3
    AEB_Status = 1;
else
    AEB_Status = 0;
end
end

== stateflow chart FCW_ROS_V1/AEB//FCA Controller1/AEB Controller/AEB Controller/AEB_Comfort ==
  note: FCW/AEB Logic
  state Default
    entry: AEBstatus = 0;
    FCWactivate = 0;
    decel = 0;
    i=0;
  state Full_Braking
  state FCW
  state Partial_Braking2
    i = 0;
    decel = 3;
  (default) -> Default
  Full_Braking -> Default [order 1] : [stop==1 || abs(TTC)>=4.2*FCWtime]
  Partial_Braking2 -> Default [order 1] : [stop==1 || abs(TTC)>=3.2*FCWtime]
  Default -> FCW : [(abs(TTC)<FCWtime) && TTC>0]{AEBstatus = 1;
      |  FCWactivate = 1;}
  FCW -> Default [order 1] : [abs(TTC)>=3.2*FCWtime]
  FCW -> (junction 74) [order 3] : {decel = decel + 0.0416; i = i+1;}
  Full_Braking -> (junction 109) [order 2] : [i<48]{decel = decel +0.0416; i = i+1;}
  (junction 74) -> (junction 105)
  (junction 109) -> (junction 110)
  (junction 105) -> FCW : [i<=72]
  (junction 110) -> Full_Braking : [i<=48]
  FCW -> Partial_Braking2 [order 2] : [i >72]{AEBstatus = 1;
      |  FCWactivate = 1;}
  Partial_Braking2 -> Full_Braking [order 2] : {AEBstatus = 2;
      |  FCWactivate = 1;}
  data: decel output; AEBstatus output; FCWactivate output; stop input; PB1decel input; PB2decel input; FBdecel input; FBtime input; PB2time input; PB1time input; FCWtime input; TTC input; i local

== stateflow chart FCW_ROS_V1/AEB//FCA Controller1/AEB Controller/AEB Controller/Chart ==
  state Default
    entry: AEBstatus = 0;
    FCWactivate = 0;
    decel = 0;
  state FCW
    entry: AEBstatus = 0;
    FCWactivate = 1;
    decel = 0;
  state Partial_Braking1
    entry: AEBstatus = 1;
    FCWactivate = 1;
    decel = PB1decel;
  state Full_Braking
    entry: AEBstatus = 3;
    FCWactivate = 1;
    decel = FBdecel;
  state Partial_Braking2
    entry: AEBstatus = 2;
    FCWactivate = 1;
    decel = PB2decel;
  (default) -> Default
  Full_Braking -> Default : [TTC > 0 && (abs(RelativeDistance) >= FCWStoppingDistance)]
  Partial_Braking2 -> Default [order 2] : [abs(RelativeDistance)>=FCWStoppingDistance && TTC >0]
  Partial_Braking1 -> Default [order 1] : [abs(RelativeDistance)>=FCWStoppingDistance && TTC >0]
  Default -> FCW : [(abs(RelativeDistance)<= 1.2*FCWStoppingDistance) && TTC>0]
  FCW -> Default [order 2] : [abs(RelativeDistance)>=FCWStoppingDistance && TTC >0]
  FCW -> Partial_Braking1 [order 1] : [TTC < 1.2 * PB1time && TTC>0]
  Partial_Braking1 -> Partial_Braking2 [order 2] : [(abs(TTC) < 1.2*PB2time) && TTC>0]
  Partial_Braking2 -> Full_Braking [order 1] : [(abs(TTC) < 1.2*FBtime) && TTC>0]
  data: TTC input; PB1time input; decel output; AEBstatus output; PB2time input; FCWactivate output; FBtime input; PB1decel input; PB2decel input; FBdecel input; stop input; FCWStoppingDistance input; RelativeDistance input

== stateflow chart FCW_ROS_V1/AEB//FCA Controller1/AEB Controller/Velocity Controller/ACC1/Chart ==
  state Velocity
    du:
    acc = pid_control(e);
    st=1;
    state acc = pid_control(e) [function]
  state Velocity1 [commented out]
    du:
    acc = pid_control(e);
    st=1;
    state acc = pid_control(e) [function] [commented out]
  state Intermediate1 [commented out]
    du:
    st=2;
  state Headway
    du:
    if (TTC~=inf)
    acc = pid_control(y);
    else
    acc=abs(pid_control(y));
    end
    st=3;
    state acc = pid_control(y) [function]
  state Headway1 [commented out]
    du:
    acc = pid_control(y);
    st=3;
    state acc = pid_control(y) [function] [commented out]
  (default) -> Velocity
  Velocity -> Headway : [RD<sd]
  Headway -> Velocity : [abs(RD)>1.05*sd]
  (default) -> Velocity1 [commented out]
  Velocity1 -> Intermediate1 [commented out] : [y<0]{i = 1; j=0; acc = 0;}
  Intermediate1 -> Velocity1 [commented out] : [y>0.2*sd && j>=100]{i=0;}
  Intermediate1 -> (junction 42) [commented out] : [0<j<101]{j=j+1;}
  Intermediate1 -> (junction 41) [commented out] : [0<i<101]{i=i+1;}
  (junction 42) -> Intermediate1 [commented out] : {acc = acc+0.05}
  (junction 41) -> Intermediate1 [commented out] : {acc = acc-0.05}
  Intermediate1 -> Headway1 [commented out] : [y<0 && i>=100]
  Headway1 -> Intermediate1 [commented out] : [y>0.2*sd]{acc=0;j=0;}
  data: e function_input double size=1; acc function_output; e function_input double size=1; acc function_output double size=1; y function_input double size=1; acc function_output; y function_input double size=1; acc function_output double size=1; i local; j local; acc output; e input; y input; st output; sd input; RD input; TTC input
